simulink model "R_I_B_block"  (R2021a)
settings: Solver=VariableStepAuto  StartTime=0.0  StopTime=10.0  RelTol=1e-3
settings Model: Creator=Nabil  LastModifiedBy=Nabil

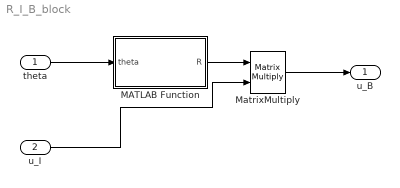
== system R_I_B_block ==
  theta : Inport
  u_I : Inport  Port=2  PortDimensions=3
  MATLAB Function : MATLAB Function  TreatAsAtomicUnit=on
  MatrixMultiply : Product  Multiplication=Matrix(*)
  u_B : Outport
  wires:
  u_I/1 -> MatrixMultiply/2
  MatrixMultiply/1 -> u_B/1
  theta/1 -> MATLAB Function/1(theta)
  MATLAB Function/1(R) -> MatrixMultiply/1

== matlab function R_I_B_block/MATLAB Function ==
  data: theta input; R output
function R = fcn(theta)

R = R_I_B(theta);
